simulink model "problem4_9"  (R2018b)
settings: Solver=VariableStepAuto  StartTime=0.0  StopTime=1000  RelTol=1e-3
values from neighbouring files (symbols this model uses):
  alphaInstant = 1    [parameters.m]
  alphaIntegral = 1    [parameters.m]
  beta0 = 0.1    [parameters.m]
  betaIntegral = 0.1    [parameters.m]
  GammaInstant = diag([300.0 50.0 10.0])    [parameters.m]
  GammaIntegral = diag([300.0 50.0 10.0])    [parameters.m]
  k0 = 5    [parameters.m]
  lambda1 = -(root1 + root2)    (= 3)    [parameters.m]
  lambda2 = root1*root2    (= 2)    [parameters.m]
  m0 = 20    [parameters.m]
  taskE = 0    [parameters.m]    (also in plot_results.m = 1)
  theta0 = [0 0 0]    [parameters.m]
  y0 = 0    [parameters.m]
  y_dot0 = 0    [parameters.m]
settings Model: Creator=cale  LastModifiedBy=cale

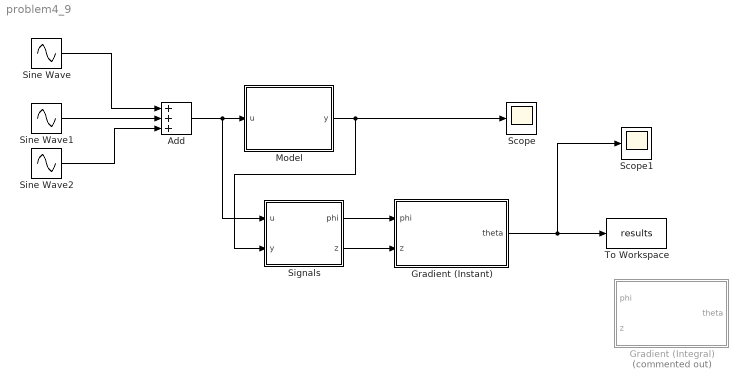
== system problem4_9 ==
  Add : Sum  Inputs=3
  Gradient (Instant) : Subsystem
  Gradient (Integral) : Subsystem  Commented=on
  Model : Subsystem
  Scope : Scope
  Scope1 : Scope
  Signals : Subsystem
  Sine Wave : Sin  Amplitude=3  Frequency=0.1  SampleTime=0
  Sine Wave1 : Sin  Frequency=5  SampleTime=0
  Sine Wave2 : Sin  Amplitude=10  Frequency=3  SampleTime=0
  To Workspace : ToWorkspace  VariableName=results  SaveFormat=Timeseries  SampleTime=-1
  wires:
  Add/1 -> Signals/1("u "), Model/1(u)
  Model/1(y) -> Signals/2("y "), Scope/1
  Signals/1(phi) -> Gradient (Instant)/1(phi)
  Gradient (Instant)/1(theta) -> Scope1/1, To Workspace/1
  Sine Wave1/1 -> Add/2
  Sine Wave/1 -> Add/1
  Sine Wave2/1 -> Add/3
  Signals/2(z) -> Gradient (Instant)/2(z)

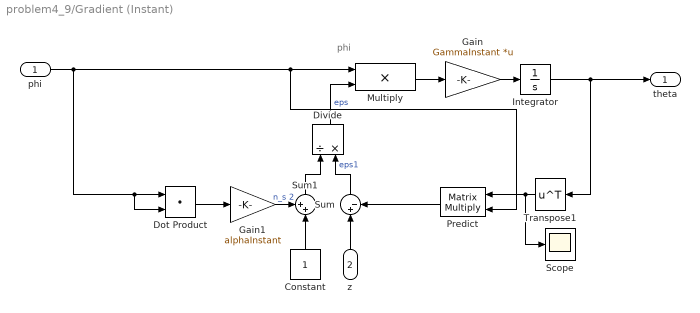
== system problem4_9/Gradient (Instant) ==
  note: phi
  phi : Inport
  z : Inport  Port=2
  Constant : Constant
  Divide : Product  Inputs=/*
  Dot Product : DotProduct  InputSameDT=on  OutDataTypeStr=Inherit: Inherit via internal rule
  Gain : Gain  Gain=GammaInstant  Multiplication=Matrix(K*u) (u vector)
  Gain1 : Gain  Gain=alphaInstant
  Integrator : Integrator  InitialCondition=theta0
  Multiply : Product
  Predict : Product  Multiplication=Matrix(*)
  Scope : Scope
  Sum : Sum  Inputs=|+-
  Sum1 : Sum  Inputs=++|
  Transpose1 : Math  Operator=transpose  SaturateOnIntegerOverflow=on
  theta : Outport
  wires:
  Multiply/1 -> Gain/1
  Gain/1 -> Integrator/1
  z/1 -> Sum/1
  Predict/1 -> Sum/2
  Sum/1 -> Divide/2  "eps1"
  Gain1/1 -> Sum1/1  "n_s 2"
  Sum1/1 -> Divide/1
  Constant/1 -> Sum1/2
  Divide/1 -> Multiply/2  "eps"
  Integrator/1 -> Transpose1/1, theta/1
  phi/1 -> Dot Product/2, Dot Product/1, Predict/2, Multiply/1
  Transpose1/1 -> Scope/1, Predict/1
  Dot Product/1 -> Gain1/1

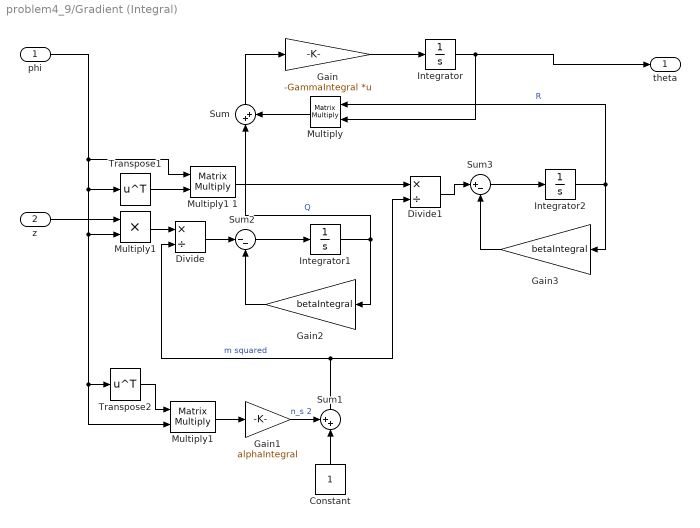
== system problem4_9/Gradient (Integral) ==
  phi : Inport
  z : Inport  Port=2
  Constant : Constant
  Divide : Product  Inputs=*/
  Divide1 : Product  Inputs=*/
  Gain : Gain  Gain=-GammaIntegral  Multiplication=Matrix(K*u) (u vector)
  Gain1 : Gain  Gain=alphaIntegral
  Gain2 : Gain  Gain=betaIntegral
  Gain3 : Gain  Gain=betaIntegral
  Integrator : Integrator  InitialCondition=theta0
  Integrator1 : Integrator
  Integrator2 : Integrator
  Multiply : Product  Multiplication=Matrix(*)
  Multiply1 : Product
  "Multiply1 " : Product  Multiplication=Matrix(*)
  Multiply1 1 : Product  Multiplication=Matrix(*)
  Sum : Sum  Inputs=|++
  Sum1 : Sum  Inputs=++|
  Sum2 : Sum  Inputs=|--
  Sum3 : Sum  Inputs=|+-
  Transpose1 : Math  Operator=transpose  SaturateOnIntegerOverflow=on
  Transpose2 : Math  Operator=transpose  SaturateOnIntegerOverflow=on
  theta : Outport
  wires:
  Gain/1 -> Integrator/1
  Gain1/1 -> Sum1/1  "n_s 2"
  Sum1/1 -> Divide/2, Divide1/2  "m squared"
  Constant/1 -> Sum1/2
  Integrator/1 -> Multiply/2, theta/1
  Transpose2/1 -> "Multiply1 "/1
  "Multiply1 "/1 -> Gain1/1
  Integrator1/1 -> Gain2/1, Sum/1  "Q"
  Sum2/1 -> Integrator1/1
  Gain2/1 -> Sum2/2
  z/1 -> Multiply1/1
  Divide/1 -> Sum2/1
  Multiply1/1 -> Divide/1
  Integrator2/1 -> Multiply/1, Gain3/1  "R"
  Gain3/1 -> Sum3/2
  Sum3/1 -> Integrator2/1
  Divide1/1 -> Sum3/1
  Sum/1 -> Gain/1
  Multiply/1 -> Sum/2
  Transpose1/1 -> Multiply1 1/2
  phi/1 -> Transpose1/1, Multiply1/2, "Multiply1 "/2, Transpose2/1, Multiply1 1/1
  Multiply1 1/1 -> Divide1/1

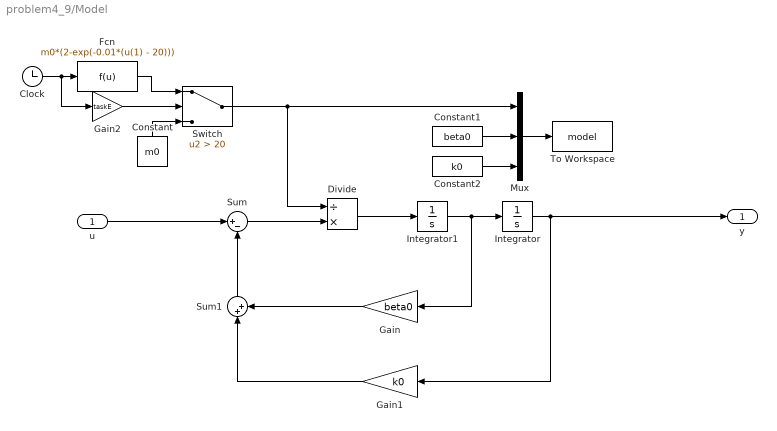
== system problem4_9/Model ==
  u : Inport
  Clock : Clock
  Constant : Constant  Value=m0
  Constant1 : Constant  Value=beta0
  Constant2 : Constant  Value=k0
  Divide : Product  Inputs=/*
  Fcn : Fcn  Expr=m0*(2-exp(-0.01*(u(1) - 20)))
  Gain : Gain  Gain=beta0
  Gain1 : Gain  Gain=k0
  Gain2 : Gain  Gain=taskE
  Integrator : Integrator  InitialCondition=y0
  Integrator1 : Integrator  InitialCondition=y_dot0
  Mux : Mux  Inputs=3
  Sum : Sum  Inputs=|+-
  Sum1 : Sum  Inputs=|++
  Switch : Switch  Criteria=u2 > Threshold  Threshold=20
  To Workspace : ToWorkspace  VariableName=model  SaveFormat=Timeseries  SampleTime=-1
  y : Outport
  wires:
  Gain1/1 -> Sum1/1
  Sum/1 -> Divide/2
  u/1 -> Sum/1
  Sum1/1 -> Sum/2
  Gain/1 -> Sum1/2
  Integrator/1 -> y/1, Gain1/1
  Divide/1 -> Integrator1/1
  Integrator1/1 -> Gain/1, Integrator/1
  Mux/1 -> To Workspace/1
  Constant1/1 -> Mux/2
  Constant2/1 -> Mux/3
  Switch/1 -> Mux/1, Divide/1
  Clock/1 -> Gain2/1, Fcn/1
  Fcn/1 -> Switch/1
  Constant/1 -> Switch/3
  Gain2/1 -> Switch/2

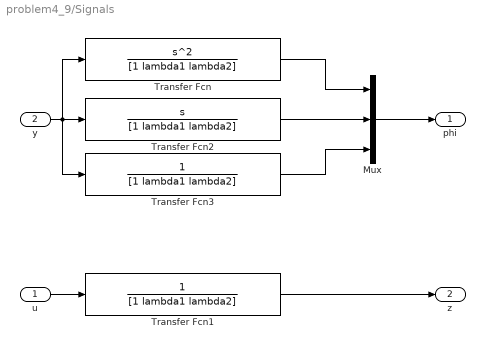
== system problem4_9/Signals ==
  "u " : Inport
  "y " : Inport  Port=2
  Mux : Mux  Inputs=3
  Transfer Fcn : TransferFcn  Numerator=[1 0 0]  Denominator=[1 lambda1 lambda2]
  Transfer Fcn1 : TransferFcn  Denominator=[1 lambda1 lambda2]
  Transfer Fcn2 : TransferFcn  Numerator=[1 0]  Denominator=[1 lambda1 lambda2]
  Transfer Fcn3 : TransferFcn  Denominator=[1 lambda1 lambda2]
  phi : Outport
  z : Outport  Port=2
  wires:
  "y "/1 -> Transfer Fcn/1, Transfer Fcn3/1, Transfer Fcn2/1
  "u "/1 -> Transfer Fcn1/1
  Transfer Fcn1/1 -> z/1
  Mux/1 -> phi/1
  Transfer Fcn/1 -> Mux/1
  Transfer Fcn2/1 -> Mux/2
  Transfer Fcn3/1 -> Mux/3
